simulink library "library"  (R2015b)
settings: Solver=VariableStepAuto  StartTime=0.0  StopTime=10.0  RelTol=1e-3
settings Model: Creator=bertram  LastModifiedBy=bertram

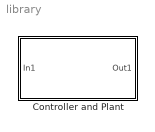
== system library ==
  Controller and Plant : Subsystem

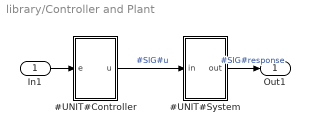
== system library/Controller and Plant ==
  In1 : Inport
  #UNIT#Controller : Subsystem  Variant=on
  #UNIT#System : Subsystem
  Out1 : Outport
  wires:
  #UNIT#System/1(out) -> Out1/1  "#SIG#response"
  In1/1 -> #UNIT#Controller/1(e)
  #UNIT#Controller/1(u) -> #UNIT#System/1(in)  "#SIG#u"

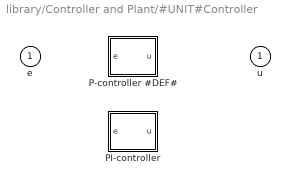
== system library/Controller and Plant/#UNIT#Controller ==
  e : Inport
  P-controller #DEF# : Subsystem  VariantControl=varsys_cond_9012b32a464bd3373daa07b1fc176436 == 1
  PI-controller : Subsystem  VariantControl=varsys_cond_9012b32a464bd3373daa07b1fc176436 == 2
  u : Outport

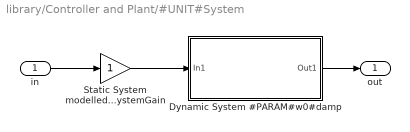
== system library/Controller and Plant/#UNIT#System ==
  in : Inport
  Dynamic System #PARAM#w0#damp : Subsystem  mask{w0=1, damp=50}
      mask prompts: w0 "Natural frequency w0 [rad/s]"; damp "Damping zeta [1]"
      mask help:
      | Dynamical system of the form
      |
      | G(s) = w0^2 / (s^2 + 2*zeta*w0*s + wo^2)
  Static System modelled by gain block #PARAM#SystemGain : Gain
  out : Outport
  wires:
  in/1 -> Static System modelled by gain block #PARAM#SystemGain/1
  Static System modelled by gain block #PARAM#SystemGain/1 -> Dynamic System #PARAM#w0#damp/1(In1)
  Dynamic System #PARAM#w0#damp/1(Out1) -> out/1

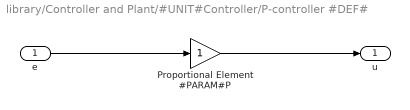
== system library/Controller and Plant/#UNIT#Controller/P-controller #DEF# ==
  e : Inport
  Proportional Element #PARAM#P : Gain
  u : Outport
  wires:
  Proportional Element #PARAM#P/1 -> u/1
  e/1 -> Proportional Element #PARAM#P/1

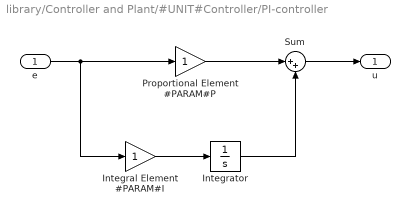
== system library/Controller and Plant/#UNIT#Controller/PI-controller ==
  e : Inport
  Integral Element #PARAM#I : Gain
  Integrator : Integrator
  Proportional Element #PARAM#P : Gain
  Sum : Sum  Inputs=|++
  u : Outport
  wires:
  Proportional Element #PARAM#P/1 -> Sum/1
  e/1 -> Integral Element #PARAM#I/1, Proportional Element #PARAM#P/1
  Sum/1 -> u/1
  Integrator/1 -> Sum/2
  Integral Element #PARAM#I/1 -> Integrator/1

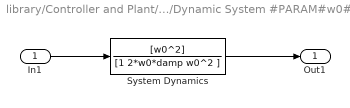
== system library/Controller and Plant/#UNIT#System/Dynamic System #PARAM#w0#damp ==
  In1 : Inport
  System Dynamics : TransferFcn  Numerator=[w0^2]  Denominator=[1 2*w0*damp w0^2 ]
  Out1 : Outport
  wires:
  System Dynamics/1 -> Out1/1
  In1/1 -> System Dynamics/1
